simulink model "Flyback_PLECS_Model_EVAL"  (R2019b)
settings: Solver=VariableStepAuto  StartTime=0.0  StopTime=.02  MaxStep=0.001e-6  RelTol=1e-3
undefined symbols (not defined in the file or in its folder): plecs
settings Model: Creator=jb  LastModifiedBy=jb
settings SolverCC: ZeroCrossAlgorithm=Adaptive
settings DebuggingCC: MaxConsecutiveZCsMsg=warning  IgnoredZcDiagnostic=none  SolverPrmCheckMsg=warning

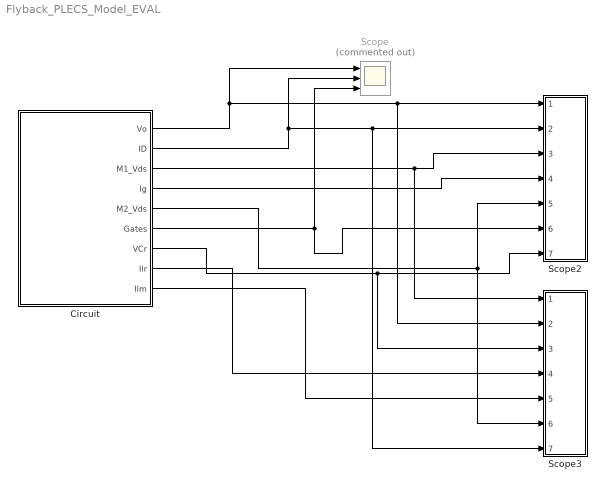
== system Flyback_PLECS_Model_EVAL ==
  Circuit : Subsystem  LoadFcn=plecs('sl', 200);  InitFcn=plecs('sl', 214);  StartFcn=plecs('sl', 208);  StopFcn=plecs('sl', 209);  mask(PlecsCircuit){PLECSData=<binary blob, 3752 chars, not shown>}
      mask prompts: PLECSData "PLECS Data (Do not delete or modify!)"
      mask init:
      | % PLACE CUSTOM INITIALIZATIONS ABOVE
      | % DO NOT REMOVE
      | plecs('sl', 215);
      | % DO NOT REMOVE
      settings: CopyFcn=plecs('sl', 203);  DeleteFcn=plecs('sl', 205);  UndoDeleteFcn=plecs('sl', 206);  PreSaveFcn=plecs('sl', 211);  PostSaveFcn=plecs('sl', 201);  NameChangeFcn=plecs('sl', 210);  DestroyFcn=plecs('sl', 207);  PreCopyFcn=plecs('sl', 216);  OpenFcn=plecs('sl', 202);  ErrorFcn=plerrorfcn
      mask Help: web(['file:///' fullfile(plecsdoc, 'creatingacircuit.html')])
      mask Display: disp('PLECS\nCircuit')
  Scope : Scope  Commented=on  NumInputPorts=3
  Scope2 : Subsystem  LoadFcn=plecs('sl', 300);  InitFcn=plecs('sl', 314);  StartFcn=plecs('sl', 308);  StopFcn=plecs('sl', 309);  mask{Settings=<binary blob, 2148 chars, not shown>}
      mask init:
      | plecs('sl', 315);
      settings: CopyFcn=plecs('sl', 303);  DeleteFcn=plecs('sl', 305);  UndoDeleteFcn=plecs('sl', 306);  PreSaveFcn=plecs('sl', 311);  NameChangeFcn=plecs('sl', 310);  DestroyFcn=plecs('sl', 307);  OpenFcn=plecs('sl', 302);  ErrorFcn=plerrorfcn
      mask Display: plot([0.1 0.9 0.9 0.1 0.1], [0.9 0.9 0.5 0.5 0.9])
  Scope3 : Subsystem  LoadFcn=plecs('sl', 300);  InitFcn=plecs('sl', 314);  StartFcn=plecs('sl', 308);  StopFcn=plecs('sl', 309);  mask{Settings=<binary blob, 1884 chars, not shown>}
      mask init:
      | plecs('sl', 315);
      settings: CopyFcn=plecs('sl', 303);  DeleteFcn=plecs('sl', 305);  UndoDeleteFcn=plecs('sl', 306);  PreSaveFcn=plecs('sl', 311);  NameChangeFcn=plecs('sl', 310);  DestroyFcn=plecs('sl', 307);  OpenFcn=plecs('sl', 302);  ErrorFcn=plerrorfcn
      mask Display: plot([0.1 0.9 0.9 0.1 0.1], [0.9 0.9 0.5 0.5 0.9])
  wires:
  Circuit/1(Vo) -> Scope/1, Scope3/2(2), Scope2/1(1)
  Circuit/2(ID) -> Scope/2, Scope3/7(7), Scope2/2(2)
  Circuit/3(M1_Vds) -> Scope3/1(1), Scope2/3(3)
  Circuit/4(Ig) -> Scope2/4(4)
  Circuit/5(M2_Vds) -> Scope2/5(5), Scope3/6(6)
  Circuit/6(Gates) -> Scope2/6(6), Scope/3
  Circuit/7(VCr) -> Scope3/3(3), Scope2/7(7)
  Circuit/8(Ilr) -> Scope3/4(4)
  Circuit/9(Ilm) -> Scope3/5(5)

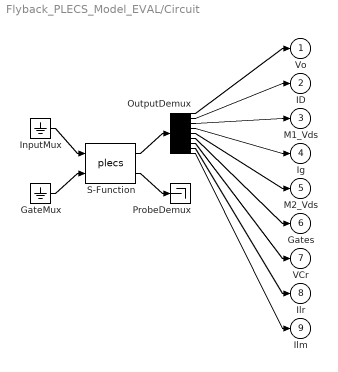
== system Flyback_PLECS_Model_EVAL/Circuit ==
  " GateMux " : Ground
  " InputMux " : Ground
  " OutputDemux " : Demux  Outputs=[ 1 2 2 1 2 1 1 1 1 ]
  " ProbeDemux " : Terminator
  " S-Function " : S-Function  FunctionName=plecs  SFunctionDeploymentMode=off  EnableBusSupport=off
  Vo : Outport  PortDimensions=1
  ID : Outport  Port=2  PortDimensions=2
  M1_Vds : Outport  Port=3  PortDimensions=2
  Ig : Outport  Port=4  PortDimensions=1
  M2_Vds : Outport  Port=5  PortDimensions=2
  Gates : Outport  Port=6  PortDimensions=1
  VCr : Outport  Port=7  PortDimensions=1
  Ilr : Outport  Port=8  PortDimensions=1
  Ilm : Outport  Port=9  PortDimensions=1
  wires:
  " InputMux "/1 -> " S-Function "/1
  " GateMux "/1 -> " S-Function "/2
  " S-Function "/1 -> " OutputDemux "/1
  " S-Function "/2 -> " ProbeDemux "/1
  " OutputDemux "/1 -> Vo/1
  " OutputDemux "/2 -> ID/1
  " OutputDemux "/3 -> M1_Vds/1
  " OutputDemux "/4 -> Ig/1
  " OutputDemux "/5 -> M2_Vds/1
  " OutputDemux "/6 -> Gates/1
  " OutputDemux "/7 -> VCr/1
  " OutputDemux "/8 -> Ilr/1
  " OutputDemux "/9 -> Ilm/1

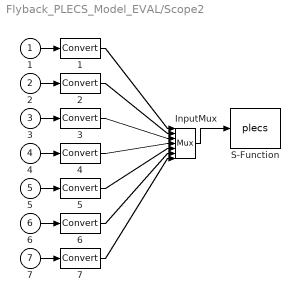
== system Flyback_PLECS_Model_EVAL/Scope2 ==
  1 : Inport
  2 : Inport  Port=2
  3 : Inport  Port=3
  4 : Inport  Port=4
  5 : Inport  Port=5
  6 : Inport  Port=6
  7 : Inport  Port=7
  " 1 " : DataTypeConversion  SaturateOnIntegerOverflow=on  RndMeth=Zero
  " 2 " : DataTypeConversion  SaturateOnIntegerOverflow=on  RndMeth=Zero
  " 3 " : DataTypeConversion  SaturateOnIntegerOverflow=on  RndMeth=Zero
  " 4 " : DataTypeConversion  SaturateOnIntegerOverflow=on  RndMeth=Zero
  " 5 " : DataTypeConversion  SaturateOnIntegerOverflow=on  RndMeth=Zero
  " 6 " : DataTypeConversion  SaturateOnIntegerOverflow=on  RndMeth=Zero
  " 7 " : DataTypeConversion  SaturateOnIntegerOverflow=on  RndMeth=Zero
  " InputMux " : Mux  Inputs=7
  " S-Function " : S-Function  FunctionName=plecs  SFunctionDeploymentMode=off  EnableBusSupport=off
  wires:
  " InputMux "/1 -> " S-Function "/1
  1/1 -> " 1 "/1
  " 1 "/1 -> " InputMux "/1
  2/1 -> " 2 "/1
  " 2 "/1 -> " InputMux "/2
  3/1 -> " 3 "/1
  " 3 "/1 -> " InputMux "/3
  4/1 -> " 4 "/1
  " 4 "/1 -> " InputMux "/4
  5/1 -> " 5 "/1
  " 5 "/1 -> " InputMux "/5
  6/1 -> " 6 "/1
  " 6 "/1 -> " InputMux "/6
  7/1 -> " 7 "/1
  " 7 "/1 -> " InputMux "/7

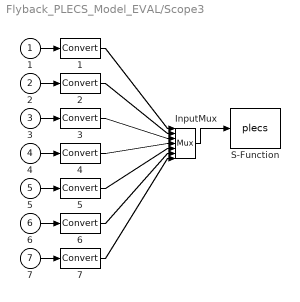
== system Flyback_PLECS_Model_EVAL/Scope3 ==
  1 : Inport
  2 : Inport  Port=2
  3 : Inport  Port=3
  4 : Inport  Port=4
  5 : Inport  Port=5
  6 : Inport  Port=6
  7 : Inport  Port=7
  " 1 " : DataTypeConversion  SaturateOnIntegerOverflow=on  RndMeth=Zero
  " 2 " : DataTypeConversion  SaturateOnIntegerOverflow=on  RndMeth=Zero
  " 3 " : DataTypeConversion  SaturateOnIntegerOverflow=on  RndMeth=Zero
  " 4 " : DataTypeConversion  SaturateOnIntegerOverflow=on  RndMeth=Zero
  " 5 " : DataTypeConversion  SaturateOnIntegerOverflow=on  RndMeth=Zero
  " 6 " : DataTypeConversion  SaturateOnIntegerOverflow=on  RndMeth=Zero
  " 7 " : DataTypeConversion  SaturateOnIntegerOverflow=on  RndMeth=Zero
  " InputMux " : Mux  Inputs=7
  " S-Function " : S-Function  FunctionName=plecs  SFunctionDeploymentMode=off  EnableBusSupport=off
  wires:
  " InputMux "/1 -> " S-Function "/1
  1/1 -> " 1 "/1
  " 1 "/1 -> " InputMux "/1
  2/1 -> " 2 "/1
  " 2 "/1 -> " InputMux "/2
  3/1 -> " 3 "/1
  " 3 "/1 -> " InputMux "/3
  4/1 -> " 4 "/1
  " 4 "/1 -> " InputMux "/4
  5/1 -> " 5 "/1
  " 5 "/1 -> " InputMux "/5
  6/1 -> " 6 "/1
  " 6 "/1 -> " InputMux "/6
  7/1 -> " 7 "/1
  " 7 "/1 -> " InputMux "/7
